simulink model "cartesianDifference"  (R2023a)
settings: Solver=ode4  StartTime=0.0  StopTime=10.0  FixedStep=dt  MaxStep=max_step_size  RelTol=relative_tolerance
settings Model: Creator=ndelurgio  LastModifiedBy=ndelurgio

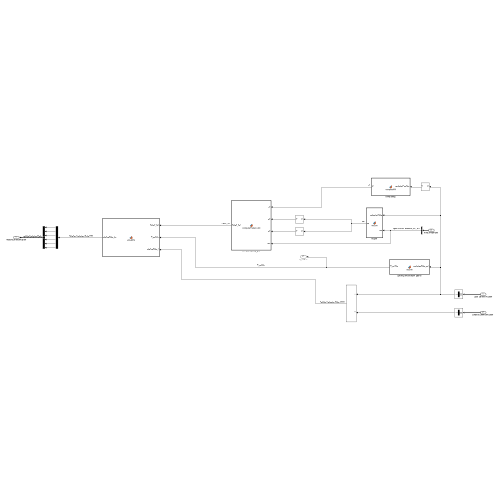
[thumbnail: Simulink's stored preview of the top-level diagram]
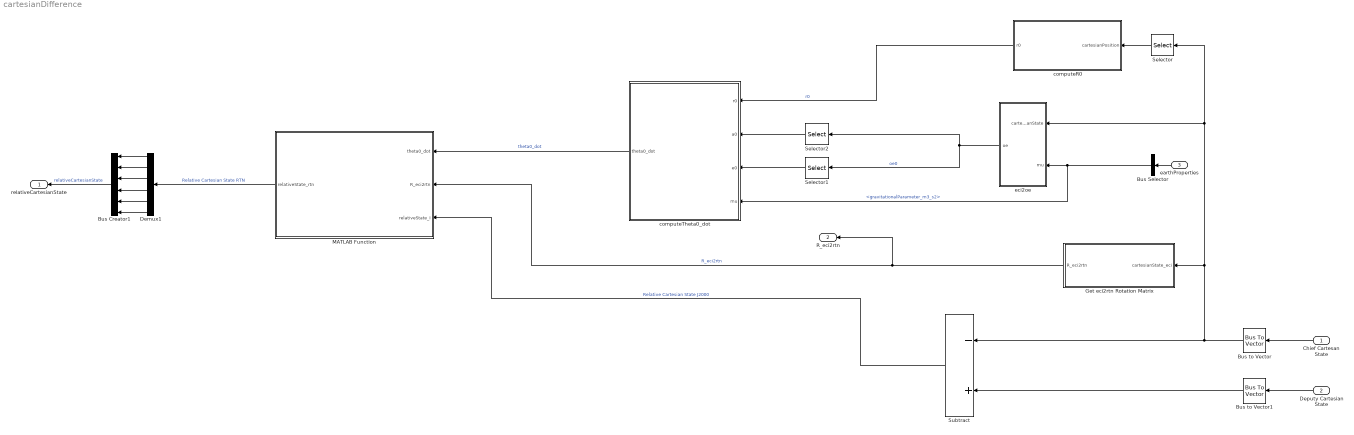
== system cartesianDifference ==
  Chief Cartesan State : Inport  OutDataTypeStr=Bus: cartesianState
  Deputy Cartesian State : Inport  Port=2  OutDataTypeStr=Bus: cartesianState
  earthProperties : Inport  Port=3  OutDataTypeStr=Bus: earthProperties
  Bus Creator1 : BusCreator  Inputs=6  OutDataTypeStr=Bus: relativeCartesianState  NonVirtualBus=on
      settings: InheritFromInputs=off
  Bus Selector : BusSelector  OutputSignals=gravitationalParameter_m3_s2
  Bus to Vector : BusToVector
  Bus to Vector1 : BusToVector
  Demux1 : Demux  Outputs=6
  Get eci2rtn Rotation Matrix : MATLAB Function  TreatAsAtomicUnit=on
  MATLAB Function : MATLAB Function  TreatAsAtomicUnit=on
  Selector : Selector  InputPortWidth=6  IndexOptions=Index vector (dialog)  Indices=1:3  OutputSizes=1
  Selector1 : Selector  InputPortWidth=6  IndexOptions=Index vector (dialog)  Indices=2  OutputSizes=1
  Selector2 : Selector  InputPortWidth=6  IndexOptions=Index vector (dialog)  Indices=1  OutputSizes=1
  Subtract : Sum  Inputs=-+
  computeR0 : MATLAB Function  TreatAsAtomicUnit=on
  computeTheta0_dot : MATLAB Function  TreatAsAtomicUnit=on
  eci2oe : MATLAB Function  TreatAsAtomicUnit=on
  relativeCartesianState : Outport  OutDataTypeStr=Bus: relativeCartesianState
  R_eci2rtn : Outport  Port=2
  wires:
  Chief Cartesan State/1 -> Bus to Vector/1
  Deputy Cartesian State/1 -> Bus to Vector1/1
  Bus to Vector/1 -> Selector/1, eci2oe/1(cartesianState), Get eci2rtn Rotation Matrix/1(cartesianState_eci), Subtract/1
  Bus to Vector1/1 -> Subtract/2
  Subtract/1 -> MATLAB Function/3(relativeState_I)  "Relative Cartesian State J2000"
  Get eci2rtn Rotation Matrix/1(R_eci2rtn) -> R_eci2rtn/1, MATLAB Function/2(R_eci2rtn)  "R_eci2rtn"
  Selector/1 -> computeR0/1(cartesianPosition)
  computeR0/1(r0) -> computeTheta0_dot/1(r0)  "r0"
  eci2oe/1(oe) -> Selector2/1, Selector1/1  "oe0"
  Selector2/1 -> computeTheta0_dot/2(a0)
  Selector1/1 -> computeTheta0_dot/3(e0)
  computeTheta0_dot/1(theta0_dot) -> MATLAB Function/1(theta0_dot)  "theta0_dot"
  MATLAB Function/1(relativeState_rtn) -> Demux1/1  "Relative Cartesian State RTN"
  earthProperties/1 -> Bus Selector/1
  Bus Selector/1 -> computeTheta0_dot/4(mu), eci2oe/2(mu)  "<gravitationalParameter_m3_s2>"
  Demux1/6 -> Bus Creator1/6
  Demux1/5 -> Bus Creator1/5
  Demux1/4 -> Bus Creator1/4
  Demux1/3 -> Bus Creator1/3
  Demux1/2 -> Bus Creator1/2
  Demux1/1 -> Bus Creator1/1
  Bus Creator1/1 -> relativeCartesianState/1  "relativeCartesianState"

== matlab function cartesianDifference/Get eci2rtn Rotation Matrix ==
  data: cartesianState_eci input; R_eci2rtn output
function R_eci2rtn  = eci2rtn(cartesianState_eci)

[~, R_eci2rtn] = eci2rtn(cartesianState_eci);

end

== matlab function cartesianDifference/computeR0 ==
  data: cartesianPosition input; r0 output
function r0  = computeR0(cartesianPosition)
r0 = computeR0(cartesianPosition);
end

== matlab function cartesianDifference/eci2oe ==
  data: cartesianState input; oe output; mu input
function oe = eci2oe(cartesianState,mu)
[oe,~,~,~] = eci2oe( cartesianState , mu );
end

== matlab function cartesianDifference/computeTheta0_dot ==
  data: r0 input; a0 input; e0 input; theta0_dot output; mu input
function theta0_dot = computeTheta0_dot(r0,a0,e0,mu)
theta0_dot = computeTheta0_dot(r0,mu,a0,e0);
end

== matlab function cartesianDifference/MATLAB Function ==
  data: theta0_dot input; R_eci2rtn input; relativeState_I input; relativeState_rtn output
function relativeState_rtn  = vI2vRTN(theta0_dot, R_eci2rtn,relativeState_I)
relativeState_rtn = vI2vRTN(relativeState_I, theta0_dot, R_eci2rtn);

end
